simulink model "CLSCIM2"  (R2016a)
settings: Solver=FixedStepDiscrete  StartTime=0.0  StopTime=3  RelTol=1e-3
libraries: powerlib x5, electricdrivelib x3, powerlib_meascontrol x2, spsDrivesDcBusModel x1
settings Model: Creator=User  LastModifiedBy=User

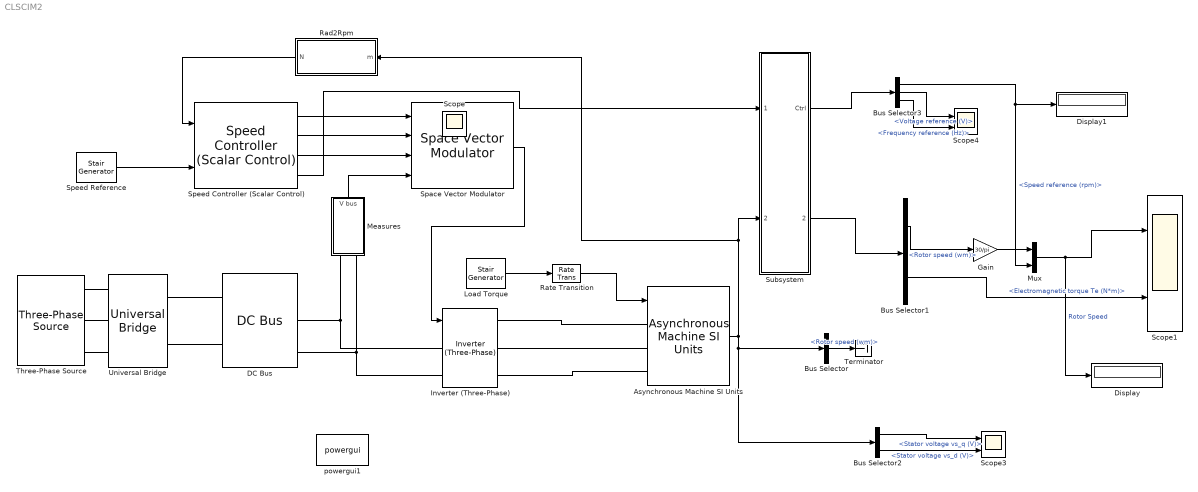
== system CLSCIM2 ==
  Asynchronous Machine SI Units : powerlib/Machines/Asynchronous Machine SI Units  RotorType=Squirrel-cage  PresetModel=No  MechanicalLoad=Torque Tm  ShowDetailedParameters=on  ReferenceFrame=Stationary  Units=SI  MeasurementBus=off  NominalParameters=[2238,220,60]  Stator=[0.435,0.002]  Rotor=[0.816,0.002]  Cage1=[0.4155 0.002066]  Cage2=[0.4168 0.0003495]  Lm=69.31e-3  Mechanical=[0.089,0.005,2]  PolePairs=2  InitialConditions=[1,0,0,0,0,0,0,0]  SimulateSaturation=off  Saturation=[14.03593122, 27.81365428, 53.79336849, 72.68890987, 97.98006896, 148.6815601, 215.7428561, 302.9841135, 428.7778367 ; 230, 322, 414, 460, 506, 552, 598, 644, 690]  LoadFlowParameters=1492000  TsPowergui=0  TsBlock=-1  IterativeModel=Trapezoidal non iterative  IterativeDiscreteModel=Trapezoidal non iterative  Pmec=0
  Bus Selector : BusSelector  OutputSignals=Mechanical.Rotor speed (wm)
  Bus Selector1 : BusSelector  OutputSignals=Mechanical.Rotor speed (wm),Mechanical.Electromagnetic torque Te (N*m)
  Bus Selector2 : BusSelector  OutputSignals=Stator measurements.Stator voltage vs_q (V),Stator measurements.Stator voltage vs_d (V)
  Bus Selector3 : BusSelector  OutputSignals=Speed reference (rpm),Voltage reference (V),Frequency reference (Hz)
  DC Bus : spsDrivesDcBusModel/DC Bus   busType=Capacitive (generic)  Ts=2e-06  capacitance=3400e-6  inductance=1e-3  Setx0=off  InitialVoltage=600  Rbrake=8  frequency=4000  activationVoltage=340  shutdownVoltage=320
  Display : Display
  Display1 : Display
  Gain : Gain  Gain=30/pi
  Inverter (Three-Phase) : electricdrivelib/Fundamental Drive Blocks/Inverter (Three-Phase)  OverrideUsingVariant=Detailed  detailLevel=Detailed  driveType=Space vector modulation  Ts=2e-6  SnubberResistance=500  SnubberCapacitance=1e-9  Device=IGBT / Diodes  Ron=1e-3  ForwardVoltages=[1.2,1.2]  GTOparameters=[1e-6,2e-6]  IGBTparameters=[1e-6,2e-6]  Measurements=All voltages and currents  converterType=Inverter  SourceFrequency=60  ReferenceFrame=Rotor  dqInductances=[8.5e-3,8.5e-3]  Inductance=8.5e-3  Ls=0  Resistance=0.2  Flux=0.175  Stator_sm=[2.01e-3,4.289e-4,4.477e-3,1.354e-3]  Stator_im=[14.85e-3,0.3027e-3]  Rotor=[9.295e-3,0.3027e-3]  Lm=10.46e-3  p=4
      settings: AttributesFormatString=%<BlockChoice>
  Load Torque : powerlib_meascontrol/Pulse & Signal Generators/Stair Generator  t=[0 0.5]  e=[0 0]  Ts=2e-06
  Measures : Subsystem
  Mux : Mux  Inputs=2
  Rad2Rpm : Subsystem
  Rate Transition : RateTransition  OutPortSampleTime=2e-06
  Scope1 : Scope  NumInputPorts=2
  Scope3 : Scope  NumInputPorts=2
  Scope4 : Scope  NumInputPorts=2
  Space Vector Modulator : electricdrivelib/Fundamental Drive Blocks/Space Vector Modulator  OverrideUsingVariant=Detailed  detailLevel=Detailed  fc_bus=50  car_freq=4500  TsMLIV=2e-6  Ts=2e-06
      settings: AttributesFormatString=%<BlockChoice>
  Speed Controller (Scalar Control) : electricdrivelib/Fundamental Drive Blocks/Speed Controller (Scalar Control)  kp=9  ki=10  vbhr=3.2  zc_time=0.4  Tsc=100e-6  bs=1800  ramp=[-1800,1800]  fc=100  ctrl_freq=[0.05,120]  ctrl_volt=[10,180]  ctrl_sat=[-30,30]  p=2  Ts=2e-06
  Speed Reference : powerlib_meascontrol/Pulse & Signal Generators/Stair Generator  t=0  e=1000  Ts=2e-06
  Subsystem : Subsystem
  Terminator : Terminator
  Three-Phase Source : powerlib/Electrical Sources/Three-Phase Source  InternalConnection=Yg  VoltagePhases=off  Voltage=220  PhaseAngle=0  Voltage_phases=[25e3 25e3 25e3]/sqrt(3)  PhaseAngles_phases=[0 -120 +120]  Frequency=60  NonIdealSource=on  SpecifyImpedance=off  Resistance=0.02  Inductance=0.05e-3  ShortCircuitLevel=100e6  BaseVoltage=25e3  XRratio=7  BusType=swing  Pref=10e3  Qref=0  Prefabc=[10e3, 10e3, 10e3]  Qrefabc=[0, 0, 0]  Qmin=-inf  Qmax=inf
  Universal Bridge : powerlib/Power Electronics/Universal Bridge  Arms=3  SnubberResistance=10e3  SnubberCapacitance=20e-9  Device=Diodes  Ron=1e-3  Lon=0  ForwardVoltages="[  0  0  ]"  ForwardVoltage=1.3  GTOparameters=[ 10e-6 , 20e-6 ]  IGBTparameters=[ 1e-6 , 2e-6 ]  Measurements=None  Measurements_2=None  converterType=Rectifier
  powergui1 : powerlib/powergui  Priority=1  SimulationMode=Discrete  SolverType=Tustin/Backward Euler (TBE)  SampleTime=2e-6  frequency=60  SPID=off  DisableSnubberDevices=off  DisableRonSwitches=off  DisableVfSwitches=off  SwTol=0  DisplayEquations=off  Interpol=off  ExternalGateDelay=off  methode=off  Ts=10  FunctionMessages=off  echomessages=off  HookPort=off  EnableUseOfTLC=off  x0status=blocks  frequencyindice=60  Pbase=100e6  ErrMax=1e-4  Iterations=50  UnitsV=kV  UnitsW=MW  buscounter=0  RestoreLinks=warning  ResistiveCurrentMeasurement=off  Frange=[0:2:500]  Ylog=off  Xlog=on  ShowGrid=off  save=off  variable=ZData  structure=0  ZoomFFT=off  StartTime=0.0  cycles=1  DisplayStyle=1  fundamental=60  FreqAxis=off  MaxFrequency=1000  frequencyindicesteady=1  RmsSteady=1  display=off
  Scope : Scope
  wires:
  Rad2Rpm/1(N) -> Speed Controller (Scalar Control)/1
  Speed Reference/1 -> Speed Controller (Scalar Control)/2
  Measures/1(V bus) -> Space Vector Modulator/4
  Speed Controller (Scalar Control)/1 -> Space Vector Modulator/1
  Speed Controller (Scalar Control)/2 -> Space Vector Modulator/2
  Speed Controller (Scalar Control)/3 -> Space Vector Modulator/3
  Rate Transition/1 -> Asynchronous Machine SI Units/1
  Space Vector Modulator/1 -> Inverter (Three-Phase)/1
  Speed Controller (Scalar Control)/4 -> Subsystem/1(Ctrl_in)
  Asynchronous Machine SI Units/1 -> Bus Selector2/1, Bus Selector/1, Rad2Rpm/1(m), Subsystem/2(Motor_in)
  Bus Selector/1 -> Terminator/1  "<Rotor speed (wm)>"
  Load Torque/1 -> Rate Transition/1
  Subsystem/2(Motor) -> Bus Selector1/1
  Bus Selector1/1 -> Gain/1  "<Rotor speed (wm)>"
  Gain/1 -> Mux/1
  Subsystem/1(Ctrl) -> Bus Selector3/1
  Bus Selector3/1 -> Display1/1, Mux/2  "<Speed reference (rpm)>"
  Mux/1 -> Scope1/1, Display/1  "Rotor Speed"
  Bus Selector1/2 -> Scope1/2  "<Electromagnetic torque Te (N*m)>"
  Bus Selector2/1 -> Scope3/1  "<Stator voltage vs_q (V)>"
  Bus Selector2/2 -> Scope3/2  "<Stator voltage vs_d (V)>"
  Bus Selector3/2 -> Scope4/1  "<Voltage reference (V)>"
  Bus Selector3/3 -> Scope4/2  "<Frequency reference (Hz)>"
  connections:
  Measures/LConn1 -- DC Bus/RConn1 -- Inverter (Three-Phase)/LConn1
  Measures/LConn2 -- Inverter (Three-Phase)/LConn2 -- DC Bus/RConn2
  Inverter (Three-Phase)/RConn1 -- Asynchronous Machine SI Units/LConn1
  Inverter (Three-Phase)/RConn2 -- Asynchronous Machine SI Units/LConn2
  Inverter (Three-Phase)/RConn3 -- Asynchronous Machine SI Units/LConn3
  Universal Bridge/RConn1 -- DC Bus/LConn1
  Universal Bridge/RConn2 -- DC Bus/LConn2
  Three-Phase Source/RConn1 -- Universal Bridge/LConn1
  Three-Phase Source/RConn2 -- Universal Bridge/LConn2
  Three-Phase Source/RConn3 -- Universal Bridge/LConn3

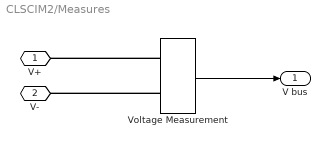
== system CLSCIM2/Measures ==
  Voltage Measurement : powerlib/Measurements/Voltage Measurement  PhasorSimulation=off  OutputType=Complex  PSBequivalent=0
  V+ : PMIOPort  Port=1  Side=Left
  V- : PMIOPort  Port=2  Side=Left
  V bus : Outport
  wires:
  Voltage Measurement/1 -> V bus/1
  connections:
  Voltage Measurement/LConn1 -- V+/RConn1
  Voltage Measurement/LConn2 -- V-/RConn1

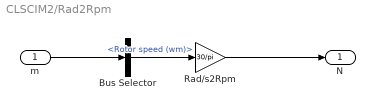
== system CLSCIM2/Rad2Rpm ==
  m : Inport
  Bus Selector : BusSelector  OutputSignals=Mechanical.Rotor speed (wm)
  Rad/s2Rpm : Gain  Gain=30/pi
  N : Outport
  wires:
  Rad/s2Rpm/1 -> N/1
  Bus Selector/1 -> Rad/s2Rpm/1  "<Rotor speed (wm)>"
  m/1 -> Bus Selector/1

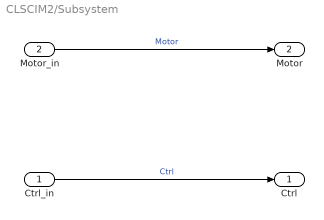
== system CLSCIM2/Subsystem ==
  Ctrl_in : Inport
  Motor_in : Inport  Port=2
  Ctrl : Outport
  Motor : Outport  Port=2
  wires:
  Ctrl_in/1 -> Ctrl/1  "Ctrl"
  Motor_in/1 -> Motor/1  "Motor"
